simulink model "dVRK_RDOBS"  (Simulink 8.5)
settings: Solver=ode4  StartTime=0.0  StopTime=length(Tm)/1000  FixedStep=0.001  RelTol=1e-3
libraries: neural x630
(part 10 of 14)

== system dVRK_RDOBS/Joint 4 NN Dyn Ident/Layer 2/Delays 1 ==
  "p{2}" : Inport  PortDimensions=100  SampleTime=0.001
      mask Display: e = 0.06;c1 = [120 230 180]/255;c2 = ([120 230 180]+0)/(256+128);c3 = ([120 230 180]+128)/(256+128);patch([0 1 1 0],[0 0 1 1],c1);patch([0 1 1 1-e 1-e 0+e],[0 0 1 1-e 0+e 0+e],c2);patch([0 0 1 1-e 0+e 0+e],[0 1 1 1-e 1-e 0+e],c3);plot([0 1 1 0 0],[0 0 1 1 0]);
  mux : Mux  Inputs=1
      mask Display: e = 0.06;c1 = [120 150 230]/255;c2 = ([120 150 230]+0)/383;c3 = ([120 150 230]+128)/383;patch([0 1 1 0],[0 0 1 1],c1);patch([0 1 1 1-e 1-e 0+e],[0 0 1 1-e 0+e 0+e],c2);patch([0 0 1 1-e 0+e 0+e],[0 1 1 1-e 1-e 0+e],c3);plot([0 1 1 0 0],[0 0 1 1 0]);disp('Mux')
  "pd{2,1}" : Outport
      mask Display: e = 0.06;c1 = [120 230 180]/255;c2 = ([120 230 180]+0)/(256+128);c3 = ([120 230 180]+128)/(256+128);patch([0 1 1 0],[0 0 1 1],c1);patch([0 1 1 1-e 1-e 0+e],[0 0 1 1-e 0+e 0+e],c2);patch([0 0 1 1-e 0+e 0+e],[0 1 1 1-e 1-e 0+e],c3);plot([0 1 1 0 0],[0 0 1 1 0]);
  wires:
  "p{2}"/1 -> mux/1
  mux/1 -> "pd{2,1}"/1

== system dVRK_RDOBS/Joint 4 NN Dyn Ident/Layer 2/LW{2,1} ==
  "ad{2,1}" : Inport  PortDimensions=100  SampleTime=0.001
      mask Display: e = 0.06;c1 = [120 230 180]/255;c2 = ([120 230 180]+0)/(256+128);c3 = ([120 230 180]+128)/(256+128);patch([0 1 1 0],[0 0 1 1],c1);patch([0 1 1 1-e 1-e 0+e],[0 0 1 1-e 0+e 0+e],c2);patch([0 0 1 1-e 0+e 0+e],[0 1 1 1-e 1-e 0+e],c3);plot([0 1 1 0 0],[0 0 1 1 0]);
  "IW{2,1}(1,:)'" : Constant  Value=[-0.079561090165099629;-1.7687788770942325;0.36356345133208506;-1.0535157417256416;-2.0903940430795802;0.42789777920118477;-0.075126161295965249;-4.6366287572324776;-0.36076993853781125;-1.0149947372059938;2.6898052556394281;0.37455263852423876;0.17928827999689495;3.0385118683155183;-3.3415194620888165;-1.3611179423168354;0.33167035668072314;0.6448201723003435;0.46989366817697126;-0.087758908318396778;-1.4491489517337821;0.17550290620778483;-0.066108407924257082;-0.18906664765386508;-0.17927240134671443;-0.20898984815612132;-0.49785666661183225;-2.6670821529191837;-0.12750106970596797;-0.12303306109063261;0.41812502558432579;0.11317959270369801;-2.0077156819039037;-1.0805257125271619;0.33060431694620424;0.10327647711033945;-1.3604236995343106;-1.548255192329679;1.5644172921905113;-0.66763705905467041;-1.6492513881925004;-0.33805353742264921;-3.0894510181058257;1.4361960853650173;1.7849820925971993;2.8201188894011753;-0.22154068534268145;-0.33529437422423813;0.047471621403046539;1.9302404971687521;0.88003221149496991;-2.0884916703217771;0.13398899162497274;-0.34378784603450752;0.63600855160749092;-0.23988203894047957;-0.26569046165817334;1.5344140557622892;-3.1606374593336639;-1.9469764921597816;4.956364108807171;2.3322841696308547;0.24732495873719557;1.1557288908898216;-0.80897342979258291;-1.5502361480312394;0.20219828755033289;0.19741903068662586;-0.084306982029344307;-0.079570311253341033;0.21665478649013747;0.10146273899180124;-0.087122256964278541;0.96455120643924241;2.2605820671860406;-0.18731343397802708;0.36712315959869402;-1.9484144824128158;2.9200594946623446;-0.064580030553620979;0.45183819150662002;1.078697553018281;0.12681388859750489;0.23300109408731248;-2.9575727576500417;0.67499924749555984;2.4245914694407906;-0.088569479432929865;-0.092861987218557429;0.23628352412232281;0.83122063826483539;0.26262766678700661;1.3075106948067434;1.5105902526821464;0.71103689914985524;0.11805145786045192;0.093962453928539635;-1.0093631828185521;0.22936111124290157;0.83850235831382258]
      mask Display: e = 0.06;c1 = [120 150 230]/255;c2 = ([120 150 230]+0)/383;c3 = ([120 150 230]+128)/383;patch([0 1 1 0],[0 0 1 1],c1);patch([0 1 1 1-e 1-e 0+e],[0 0 1 1-e 0+e 0+e],c2);patch([0 0 1 1-e 0+e 0+e],[0 1 1 1-e 1-e 0+e],c3);plot([0 1 1 0 0],[0 0 1 1 0]);disp('weights');
  Mux : Mux  Inputs=1
      mask Display: e = 0.06;c1 = [120 150 230]/255;c2 = ([120 150 230]+0)/383;c3 = ([120 150 230]+128)/383;patch([0 1 1 0],[0 0 1 1],c1);patch([0 1 1 1-e 1-e 0+e],[0 0 1 1-e 0+e 0+e],c2);patch([0 0 1 1-e 0+e 0+e],[0 1 1 1-e 1-e 0+e],c3);plot([0 1 1 0 0],[0 0 1 1 0]);disp('Mux');
  dotprod1 : neural/Weight Functions/dotprod
  "lz{2,1}" : Outport
      mask Display: e = 0.06;c1 = [120 230 180]/255;c2 = ([120 230 180]+0)/(256+128);c3 = ([120 230 180]+128)/(256+128);patch([0 1 1 0],[0 0 1 1],c1);patch([0 1 1 1-e 1-e 0+e],[0 0 1 1-e 0+e 0+e],c2);patch([0 0 1 1-e 0+e 0+e],[0 1 1 1-e 1-e 0+e],c3);plot([0 1 1 0 0],[0 0 1 1 0]);
  wires:
  "IW{2,1}(1,:)'"/1 -> dotprod1/1
  "ad{2,1}"/1 -> dotprod1/2
  dotprod1/1 -> Mux/1
  Mux/1 -> "lz{2,1}"/1

== system dVRK_RDOBS/Joint 5 NN Dyn Ident/Layer 1/Delays 1 ==
  "p{1}" : Inport  PortDimensions=12  SampleTime=0.001
      mask Display: e = 0.06;c1 = [120 230 180]/255;c2 = ([120 230 180]+0)/(256+128);c3 = ([120 230 180]+128)/(256+128);patch([0 1 1 0],[0 0 1 1],c1);patch([0 1 1 1-e 1-e 0+e],[0 0 1 1-e 0+e 0+e],c2);patch([0 0 1 1-e 0+e 0+e],[0 1 1 1-e 1-e 0+e],c3);plot([0 1 1 0 0],[0 0 1 1 0]);
  mux : Mux  Inputs=1
      mask Display: e = 0.06;c1 = [120 150 230]/255;c2 = ([120 150 230]+0)/383;c3 = ([120 150 230]+128)/383;patch([0 1 1 0],[0 0 1 1],c1);patch([0 1 1 1-e 1-e 0+e],[0 0 1 1-e 0+e 0+e],c2);patch([0 0 1 1-e 0+e 0+e],[0 1 1 1-e 1-e 0+e],c3);plot([0 1 1 0 0],[0 0 1 1 0]);disp('Mux')
  "pd{1,1}" : Outport
      mask Display: e = 0.06;c1 = [120 230 180]/255;c2 = ([120 230 180]+0)/(256+128);c3 = ([120 230 180]+128)/(256+128);patch([0 1 1 0],[0 0 1 1],c1);patch([0 1 1 1-e 1-e 0+e],[0 0 1 1-e 0+e 0+e],c2);patch([0 0 1 1-e 0+e 0+e],[0 1 1 1-e 1-e 0+e],c3);plot([0 1 1 0 0],[0 0 1 1 0]);
  wires:
  "p{1}"/1 -> mux/1
  mux/1 -> "pd{1,1}"/1
